simulink model "DT_SigmaDelta"  (Simulink 7.9)
settings: Solver=VariableStepDiscrete  StartTime=0.0  StopTime=1  RelTol=1e-6
PreLoadFcn:
  | load one_stage.mat
undefined symbols (not defined in the file or in its folder): DiscIntNeverNeededParam
libraries: dspmlti4 x21, simulink x3, dspvision x1
(part 12 of 13)

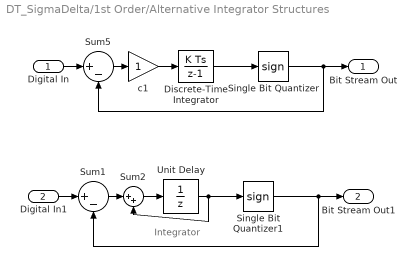
== system DT_SigmaDelta/1st Order/Alternative Integrator Structures ==
  note: Integrator
  Digital In : Inport
  Digital In1 : Inport  Port=2
  Discrete-Time Integrator : DiscreteIntegrator  SampleTime=1/(48e3*64)  UpperSaturationLimit=1  LowerSaturationLimit=-1  ICPrevOutput=DiscIntNeverNeededParam  ICPrevScaledInput=DiscIntNeverNeededParam
  Single Bit Quantizer : Signum  SampleTime=1/(48e3*64)
  Single Bit Quantizer1 : Signum  SampleTime=1/(48e3*64)
  Sum1 : Sum  Inputs=|+-  AccumDataTypeStr=double  SampleTime=1/(48e3*64)
  Sum2 : Sum  Inputs=|++
  Sum5 : Sum  Inputs=|+-  AccumDataTypeStr=double  SampleTime=1/(48e3*64)
  Unit Delay : UnitDelay  SampleTime=1/(48e3*64)
  c1 : Gain  SampleTime=1/(48e3*64)
  Bit Stream Out : Outport  OutDataTypeStr=double
  Bit Stream Out1 : Outport  Port=2  OutDataTypeStr=double
  wires:
  Digital In/1 -> Sum5/1
  Single Bit Quantizer/1 -> Bit Stream Out/1, Sum5/2
  Discrete-Time Integrator/1 -> Single Bit Quantizer/1
  Sum5/1 -> c1/1
  c1/1 -> Discrete-Time Integrator/1
  Sum1/1 -> Sum2/1
  Digital In1/1 -> Sum1/1
  Single Bit Quantizer1/1 -> Bit Stream Out1/1, Sum1/2
  Unit Delay/1 -> Single Bit Quantizer1/1, Sum2/2
  Sum2/1 -> Unit Delay/1
